simulink model "NPSS_TTECTrA"  (Simulink 7.5)
settings: Solver=FixedStepDiscrete  StartTime=0.0  StopTime=20  FixedStep=0.02  RelTol=1e-3
undefined symbols (not defined in the file or in its folder): DiscIntNeverNeededParam
libraries: simulink x2
settings Model: Creator=jcsank  LastModifiedBy=jcsank

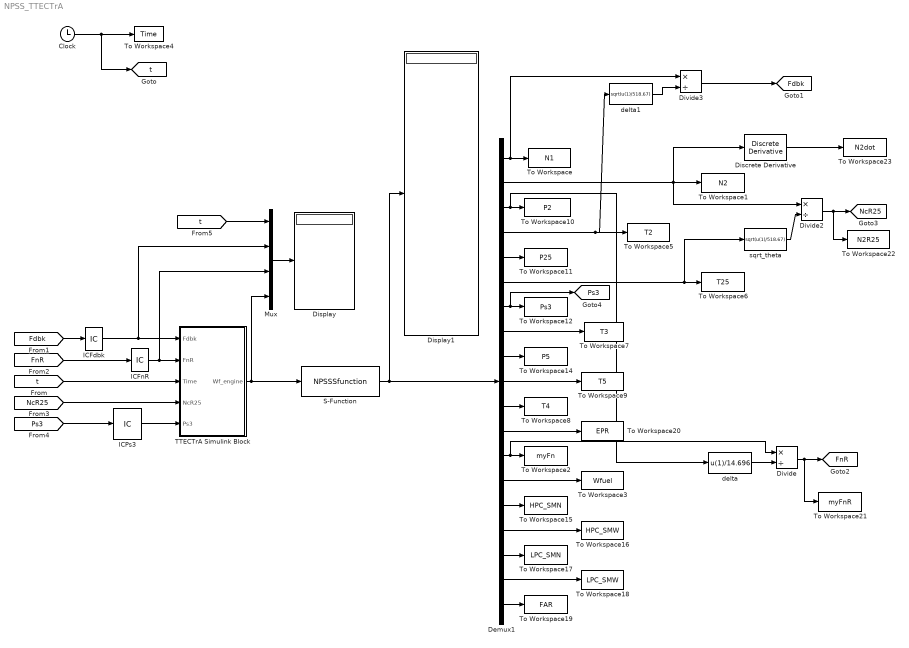
== system NPSS_TTECTrA ==
  Clock : Clock
      settings: Decimation=10
  Demux1 : Demux  Outputs=19
  Discrete Derivative : simulink/Discrete/Discrete Derivative  SystemSampleTime=-1  gainval=1.0  ICPrevScaledInput=0.0  OutMin=[]  OutMax=[]  OutDataType=fixdt(1, 16)  OutScaling=2^-10  DoSatur=off
  Display : Display
  Display1 : Display
  Divide : Product  Inputs=*/
  Divide2 : Product  Inputs=*/
  Divide3 : Product  Inputs=*/
  ICFdbk : InitialCondition  Value=4546.886
  ICFnR : InitialCondition  Value=20944.236
  ICPs3 : InitialCondition  Value=313.2783
  Mux : Mux
  S-Function : S-Function  FunctionName=NPSSSfunction  Parameters='150_PAX_Sfunction.config'  EnableBusSupport=off
  TTECTrA Simulink Block : Subsystem
  To Workspace : ToWorkspace  VariableName=N1  SampleTime=-1  SaveFormat=Array
  To Workspace1 : ToWorkspace  VariableName=N2  SampleTime=-1  SaveFormat=Array
  To Workspace10 : ToWorkspace  VariableName=P2  SampleTime=-1  SaveFormat=Array
  To Workspace11 : ToWorkspace  VariableName=P25  SampleTime=-1  SaveFormat=Array
  To Workspace12 : ToWorkspace  VariableName=Ps3  SampleTime=-1  SaveFormat=Array
  To Workspace14 : ToWorkspace  VariableName=P5  SampleTime=-1  SaveFormat=Array
  To Workspace15 : ToWorkspace  VariableName=HPC_SMN  SampleTime=-1  SaveFormat=Array
  To Workspace16 : ToWorkspace  VariableName=HPC_SMW  SampleTime=-1  SaveFormat=Array
  To Workspace17 : ToWorkspace  VariableName=LPC_SMN  SampleTime=-1  SaveFormat=Array
  To Workspace18 : ToWorkspace  VariableName=LPC_SMW  SampleTime=-1  SaveFormat=Array
  To Workspace19 : ToWorkspace  VariableName=FAR  SampleTime=-1  SaveFormat=Array
  To Workspace2 : ToWorkspace  VariableName=myFn  SampleTime=-1  SaveFormat=Array
  To Workspace20 : ToWorkspace  VariableName=EPR  SampleTime=-1  SaveFormat=Array
  To Workspace21 : ToWorkspace  VariableName=myFnR  SampleTime=-1  SaveFormat=Array
  To Workspace22 : ToWorkspace  VariableName=N2R25  SampleTime=-1  SaveFormat=Array
  To Workspace23 : ToWorkspace  VariableName=N2dot  SampleTime=-1  SaveFormat=Array
  To Workspace3 : ToWorkspace  VariableName=Wfuel  SampleTime=-1  SaveFormat=Array
  To Workspace4 : ToWorkspace  VariableName=Time  SampleTime=-1  SaveFormat=Array
  To Workspace5 : ToWorkspace  VariableName=T2  SampleTime=-1  SaveFormat=Array
  To Workspace6 : ToWorkspace  VariableName=T25  SampleTime=-1  SaveFormat=Array
  To Workspace7 : ToWorkspace  VariableName=T3  SampleTime=-1  SaveFormat=Array
  To Workspace8 : ToWorkspace  VariableName=T4  SampleTime=-1  SaveFormat=Array
  To Workspace9 : ToWorkspace  VariableName=T5  SampleTime=-1  SaveFormat=Array
  delta : Fcn  Expr=u(1)/14.696
  delta1 : Fcn  Expr=sqrt(u(1)/518.67)
  sqrt_theta : Fcn  Expr=sqrt(u(1)/518.67)
  tag scope: Fdbk=global, FnR=global, NcR25=global, Ps3=global, t=global
  wires:
  S-Function/1 -> Demux1/1, Display1/1
  Clock/1 -> [t], To Workspace4/1
  TTECTrA Simulink Block/1(Wf_engine) -> Mux/4, S-Function/1
  [t] -> TTECTrA Simulink Block/3(Time)
  [Fdbk] -> ICFdbk/1
  [FnR] -> ICFnR/1
  [NcR25] -> TTECTrA Simulink Block/4(NcR25)
  Divide/1 -> [FnR], To Workspace21/1
  delta/1 -> Divide/2
  Divide2/1 -> [NcR25], To Workspace22/1
  Discrete Derivative/1 -> To Workspace23/1
  [t] -> Mux/1
  Mux/1 -> Display/1
  [Ps3] -> ICPs3/1
  Demux1/1 -> To Workspace/1, Divide3/1
  Demux1/2 -> To Workspace1/1, Discrete Derivative/1, Divide2/1
  Demux1/3 -> To Workspace10/1, delta/1
  Demux1/4 -> To Workspace5/1, delta1/1
  Demux1/5 -> To Workspace11/1
  Demux1/6 -> To Workspace6/1, sqrt_theta/1
  Demux1/7 -> To Workspace12/1, [Ps3]
  Demux1/8 -> To Workspace7/1
  Demux1/10 -> To Workspace9/1
  Demux1/9 -> To Workspace14/1
  Demux1/11 -> To Workspace8/1
  Demux1/12 -> To Workspace20/1
  Demux1/13 -> To Workspace2/1, Divide/1
  Demux1/14 -> To Workspace3/1
  Demux1/15 -> To Workspace15/1
  Demux1/16 -> To Workspace16/1
  Demux1/17 -> To Workspace17/1
  Demux1/18 -> To Workspace18/1
  Demux1/19 -> To Workspace19/1
  sqrt_theta/1 -> Divide2/2
  delta1/1 -> Divide3/2
  Divide3/1 -> [Fdbk]
  ICFdbk/1 -> TTECTrA Simulink Block/1(Fdbk), Mux/2
  ICPs3/1 -> TTECTrA Simulink Block/5(Ps3)
  ICFnR/1 -> TTECTrA Simulink Block/2("FnR "), Mux/3

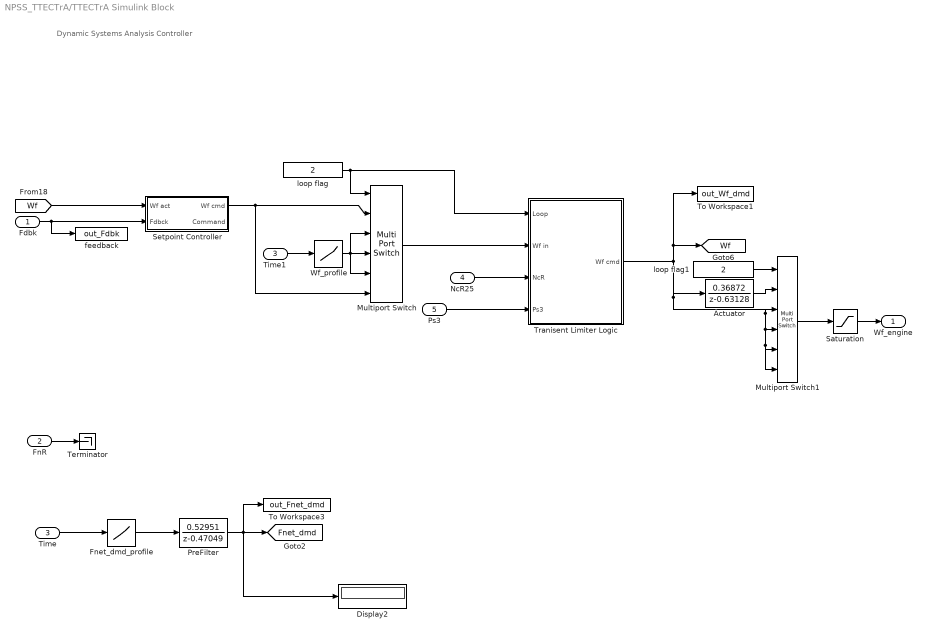
== system NPSS_TTECTrA/TTECTrA Simulink Block ==
  note: Dynamic Systems Analysis Controller
  Fdbk : Inport
  "FnR " : Inport  Port=2
  Time : Inport  Port=3
  NcR25 : Inport  Port=4
  Ps3 : Inport  Port=5
  Actuator : DiscreteTransferFcn  Numerator=[0.36872]  Denominator="[1    -0.63128]"  InitialStates=[1.9401]  SampleTime=-1
  Display2 : Display
  Fnet_dmd_profile : Lookup  InputValues="[0  10  16  20]"  Table="[30000  30000  30000  30000]"  SampleTime=0.02
  Multiport Switch : MultiPortSwitch  Inputs=5  zeroidx=off  SampleTime=0.02
  Multiport Switch1 : MultiPortSwitch  Inputs=5  zeroidx=off  SampleTime=0.02
  PreFilter : DiscreteTransferFcn  Numerator=[0.52951]  Denominator="[1    -0.47049]"  InitialStates=[30000]  SampleTime=-1
  Saturation : Saturate  UpperLimit=9999  LowerLimit=0
  Setpoint Controller : Subsystem
  Terminator : Terminator
  Time1 : InportShadow  Port=3
  To Workspace1 : ToWorkspace  VariableName=out_Wf_dmd  SampleTime=-1  SaveFormat=Array
  To Workspace3 : ToWorkspace  VariableName=out_Fnet_dmd  SampleTime=-1  SaveFormat=Array
  Tranisent Limiter Logic : Subsystem
  Wf_profile : Lookup  InputValues="[0  10  16  20]"  Table="[1.9401      1.9401      1.2316      1.2316]"  SampleTime=0.02
  feedback : ToWorkspace  VariableName=out_Fdbk  SampleTime=-1  SaveFormat=Array
  loop flag : Constant  Value=2
  loop flag1 : Constant  Value=2
  Wf_engine : Outport
  tag scope: Fnet_dmd=global, Wf=global
  wires:
  [Wf] -> Setpoint Controller/1(Wf act)
  Fdbk/1 -> feedback/1, Setpoint Controller/2(Fdbck)
  Time/1 -> Fnet_dmd_profile/1
  NcR25/1 -> Tranisent Limiter Logic/3(NcR)
  Fnet_dmd_profile/1 -> PreFilter/1
  PreFilter/1 -> [Fnet_dmd], To Workspace3/1, Display2/1
  Saturation/1 -> Wf_engine/1
  Multiport Switch1/1 -> Saturation/1
  loop flag1/1 -> Multiport Switch1/1
  Ps3/1 -> Tranisent Limiter Logic/4(Ps3)
  Time1/1 -> Wf_profile/1
  loop flag/1 -> Tranisent Limiter Logic/1(Loop), Multiport Switch/1
  Multiport Switch/1 -> Tranisent Limiter Logic/2(Wf in)
  Wf_profile/1 -> Multiport Switch/4, Multiport Switch/3, Multiport Switch/5
  Setpoint Controller/1(Wf cmd) -> Multiport Switch/2, Multiport Switch/6
  "FnR "/1 -> Terminator/1
  Actuator/1 -> Multiport Switch1/2
  Tranisent Limiter Logic/1(Wf cmd) -> [Wf], To Workspace1/1, Actuator/1, Multiport Switch1/3, Multiport Switch1/4, Multiport Switch1/5, Multiport Switch1/6

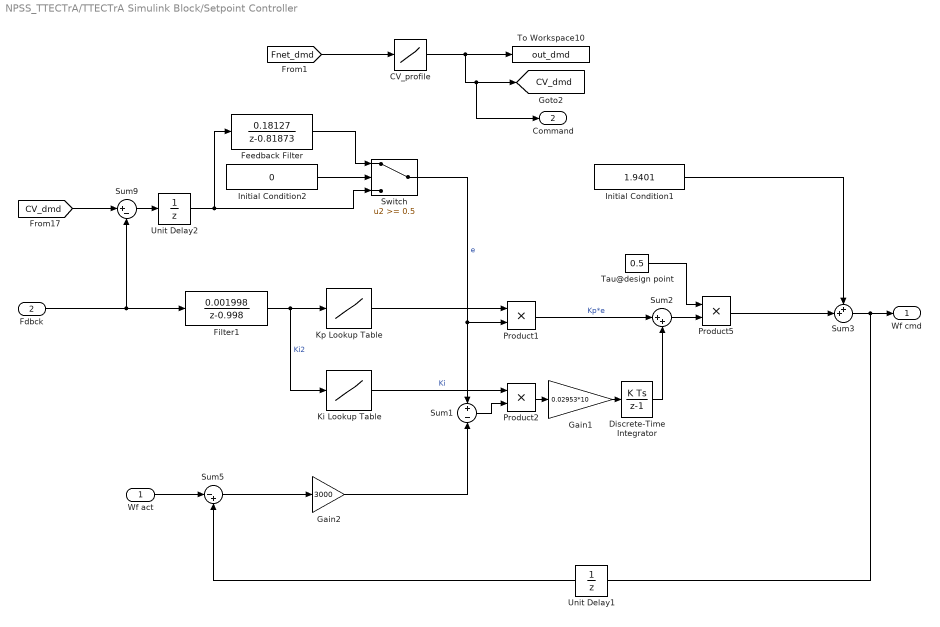
== system NPSS_TTECTrA/TTECTrA Simulink Block/Setpoint Controller ==
  Wf act : Inport
  Fdbck : Inport  Port=2
  CV_profile : Lookup  InputValues="[10000  10952  11905  12857  13810  14762  15714  16667  17619  18571  19524  20476  21429  22381  23333  24286  25238  26190  26500]"  Table="[3351.08        3485.18        3617.09        3736.41        3841.09         3946.6         4047.8        4147.36        4243.83        4334.02        4423.46         4508.7        4586.42        4663.34        4743.77        4827.12        4910.63         4994.1        5027.53]"  LookUpMeth=Interpolation-Use End Values  SampleTime=0.02
  Discrete-Time Integrator : DiscreteIntegrator  SampleTime=-1  ICPrevOutput=DiscIntNeverNeededParam  ICPrevScaledInput=DiscIntNeverNeededParam
  Feedback Filter : DiscreteTransferFcn  Numerator=[0.18127]  Denominator="[1    -0.81873]"  SampleTime=0.02
  Filter1 : DiscreteTransferFcn  Numerator=[0.001998]  Denominator="[1      -0.998]"  SampleTime=0.02
  Gain1 : Gain  Gain=0.02953*10
  Gain2 : Gain  Gain=3000
  Initial Condition1 : Constant  Value=1.9401
  Initial Condition2 : Constant  Value=0
  Ki Lookup Table : Lookup_n-D  NumberOfTableDimensions=1  BreakpointsForDimension1="[1000  5000]"  Table="[1  2]"  SampleTime=0.02  RndMeth=Simplest  InputSameDT=on
  Kp Lookup Table : Lookup_n-D  NumberOfTableDimensions=1  BreakpointsForDimension1="[1000  5000]"  Table="[1  2]"  SampleTime=0.02  RndMeth=Simplest  InputSameDT=on
  Product1 : Product  SampleTime=0.02  RndMeth=Zero
  Product2 : Product  RndMeth=Zero
  Product5 : Product  SampleTime=0.02  RndMeth=Zero
  Sum1 : Sum  Inputs=+|-
  Sum2 : Sum  Inputs=|++  SampleTime=0.02
  Sum3 : Sum  Inputs=++|  SampleTime=0.02
  Sum5 : Sum  Inputs=|-+
  Sum9 : Sum  Inputs=|+-  SampleTime=0.02
  Switch : Switch  Threshold=0.5  SampleTime=0.02
  Tau@design point : Constant  Value=0.5
  To Workspace10 : ToWorkspace  VariableName=out_dmd  SampleTime=-1  SaveFormat=Array
  Unit Delay1 : UnitDelay  SampleTime=-1
  Unit Delay2 : UnitDelay  SampleTime=-1
  Wf cmd : Outport
  Command : Outport  Port=2
  tag scope: CV_dmd=global
  wires:
  Tau@design point/1 -> Product5/1
  Product1/1 -> Sum2/1  "Kp*e"
  Product2/1 -> Gain1/1
  Sum9/1 -> Unit Delay2/1
  [CV_dmd] -> Sum9/1
  Wf act/1 -> Sum5/1
  Sum5/1 -> Gain2/1
  Switch/1 -> Product1/2, Sum1/1  "e"
  Sum1/1 -> Product2/2
  Sum2/1 -> Product5/2
  Gain2/1 -> Sum1/2
  Sum3/1 -> Wf cmd/1, Unit Delay1/1
  Initial Condition1/1 -> Sum3/1
  Product5/1 -> Sum3/2
  Gain1/1 -> Discrete-Time Integrator/1
  Discrete-Time Integrator/1 -> Sum2/2
  Ki Lookup Table/1 -> Product2/1  "Ki"
  Fdbck/1 -> Sum9/2, Filter1/1
  CV_profile/1 -> To Workspace10/1, [CV_dmd], Command/1
  [Fnet_dmd] -> CV_profile/1
  Kp Lookup Table/1 -> Product1/1
  Filter1/1 -> Ki Lookup Table/1, Kp Lookup Table/1  "Ki2"
  Initial Condition2/1 -> Switch/2
  Feedback Filter/1 -> Switch/1
  Unit Delay1/1 -> Sum5/2
  Unit Delay2/1 -> Switch/3, Feedback Filter/1

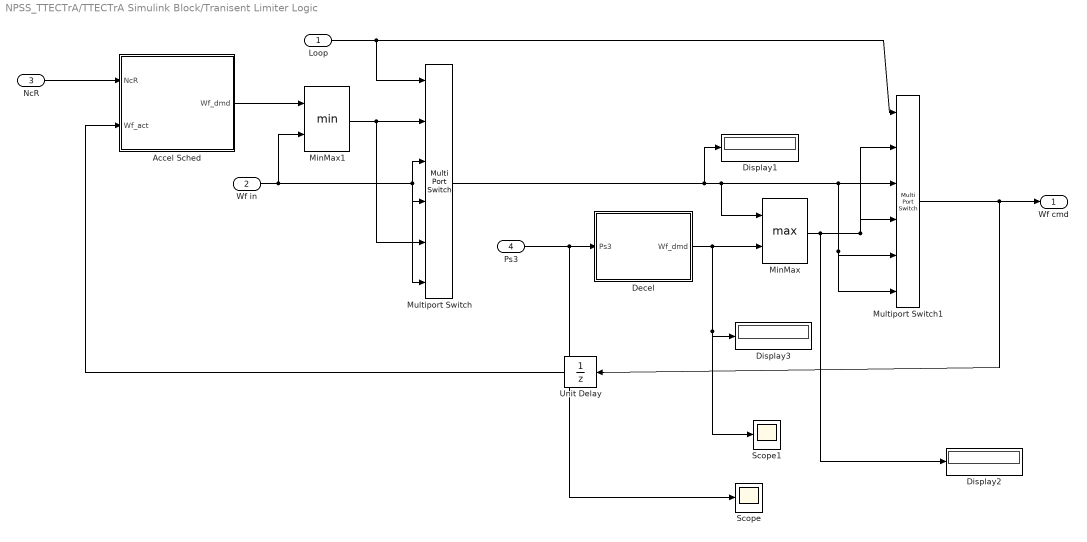
== system NPSS_TTECTrA/TTECTrA Simulink Block/Tranisent Limiter Logic ==
  Loop : Inport
  Wf in : Inport  Port=2
  NcR : Inport  Port=3
  Ps3 : Inport  Port=4
  Accel Sched : Subsystem
  Decel : Subsystem
  Display1 : Display
  Display2 : Display
  Display3 : Display
  MinMax : MinMax  Function=max  Inputs=2  SampleTime=0.02
  MinMax1 : MinMax  Inputs=2  SampleTime=0.02
  Multiport Switch : MultiPortSwitch  Inputs=5  zeroidx=off  SampleTime=0.02
  Multiport Switch1 : MultiPortSwitch  Inputs=5  zeroidx=off  SampleTime=0.02
  Scope : Scope
  Scope1 : Scope
  Unit Delay : UnitDelay  SampleTime=-1
  Wf cmd : Outport
  wires:
  NcR/1 -> Accel Sched/1(NcR)
  Unit Delay/1 -> Accel Sched/2(Wf_act)
  Loop/1 -> Multiport Switch/1, Multiport Switch1/1
  Accel Sched/1(Wf_dmd) -> MinMax1/1
  Wf in/1 -> Multiport Switch/4, Multiport Switch/3, Multiport Switch/6, MinMax1/2
  Ps3/1 -> Decel/1(Ps3), Scope/1
  Multiport Switch1/1 -> Unit Delay/1, Wf cmd/1
  MinMax/1 -> Multiport Switch1/4, Multiport Switch1/2, Display2/1
  Multiport Switch/1 -> MinMax/1, Multiport Switch1/3, Multiport Switch1/5, Multiport Switch1/6, Display1/1
  Decel/1(Wf_dmd) -> MinMax/2, Display3/1, Scope1/1
  MinMax1/1 -> Multiport Switch/2, Multiport Switch/5

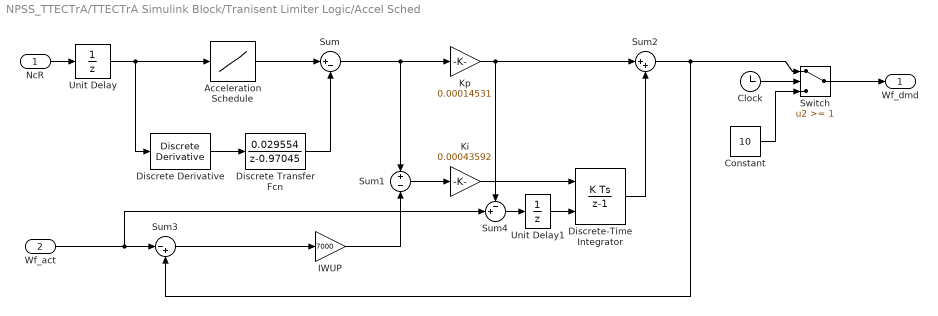
== system NPSS_TTECTrA/TTECTrA Simulink Block/Tranisent Limiter Logic/Accel Sched ==
  NcR : Inport
  Wf_act : Inport  Port=2
  Acceleration Schedule : Lookup  InputValues="[7500  11000]"  Table="[150  150]"  SampleTime=0.02
  Clock : Clock
      settings: Decimation=10
  Constant : Constant  Value=10  OutDataType=fixdt(1, 16)  OutScaling=2^0
  Discrete Derivative : simulink/Discrete/Discrete Derivative  SystemSampleTime=-1  gainval=1.0  ICPrevScaledInput=0  OutMin=[]  OutMax=[]  OutDataType=fixdt(1, 16)  OutScaling=2^-10  DoSatur=off
  Discrete Transfer Fcn : DiscreteTransferFcn  Numerator=[0.029554]  Denominator="[1    -0.97045]"  SampleTime=0.02
  Discrete-Time Integrator : DiscreteIntegrator  InitialConditionSource=external  SampleTime=0.02  ICPrevOutput=DiscIntNeverNeededParam  ICPrevScaledInput=DiscIntNeverNeededParam
  IWUP : Gain  Gain=7000
  Ki : Gain  Gain=0.00043592
  Kp : Gain  Gain=0.00014531  SampleTime=0.02
  Sum : Sum  Inputs=|+-  SampleTime=0.02
  Sum1 : Sum  Inputs=+|-
  Sum2 : Sum  Inputs=|++  SampleTime=0.02
  Sum3 : Sum  Inputs=|-+
  Sum4 : Sum  Inputs=-+|  SampleTime=0.02
  Switch : Switch  Threshold=1  OutDataType=fixdt(1, 16)  OutScaling=2^0
  Unit Delay : UnitDelay  SampleTime=-1
  Unit Delay1 : UnitDelay  SampleTime=-1
  Wf_dmd : Outport
  wires:
  NcR/1 -> Unit Delay/1
  Discrete Derivative/1 -> Discrete Transfer Fcn/1
  Acceleration Schedule/1 -> Sum/1
  Discrete Transfer Fcn/1 -> Sum/2
  Sum/1 -> Sum1/1, Kp/1
  Sum1/1 -> Ki/1
  Kp/1 -> Sum4/1, Sum2/1
  Sum2/1 -> Sum3/2, Switch/1
  Ki/1 -> Discrete-Time Integrator/1
  Discrete-Time Integrator/1 -> Sum2/2
  IWUP/1 -> Sum1/2
  Sum3/1 -> IWUP/1
  Wf_act/1 -> Sum4/2, Sum3/1
  Sum4/1 -> Unit Delay1/1
  Unit Delay/1 -> Discrete Derivative/1, Acceleration Schedule/1
  Unit Delay1/1 -> Discrete-Time Integrator/2
  Clock/1 -> Switch/2
  Constant/1 -> Switch/3
  Switch/1 -> Wf_dmd/1

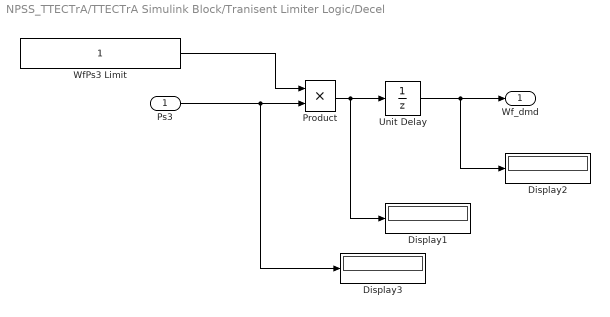
== system NPSS_TTECTrA/TTECTrA Simulink Block/Tranisent Limiter Logic/Decel ==
  Ps3 : Inport
  Display1 : Display
  Display2 : Display
  Display3 : Display
  Product : Product  RndMeth=Zero
  Unit Delay : UnitDelay  X0=1.9401  SampleTime=-1
  WfPs3 Limit : Constant
  Wf_dmd : Outport
  wires:
  Ps3/1 -> Product/2, Display3/1
  WfPs3 Limit/1 -> Product/1
  Product/1 -> Unit Delay/1, Display1/1
  Unit Delay/1 -> Wf_dmd/1, Display2/1
